simulink model "testrig_Sedan_Hamba_Parts"  (R2026a)
settings: Solver=VariableStepAuto
model workspace (MAT data in the model file):
  smiData : object (value not decoded)
undefined symbols (not defined in the file): Visual, X, Y, Z
libraries: sm_lib x9, Sedan_Hamba_Parts x5, Driver_Human x1, nesl_utility x1, SteeringWheel_Sedan x1
Description:
  | Copyright 2020-2026 The MathWorks, Inc.
settings Model: Creator=smiller  LastModifiedBy=smiller
settings DataIOCC: SignalLoggingName=logsout_testrig_Sedan_Hamba_Parts
settings SimscapeCC: SimscapeNominalValues="[{\"value\":\"1\",\"unit\":\"A\"},{\"value\":\"1\",\"unit\":\"bar\"},{\"value\":\"1\",\"unit\":\"cm^2\"},{\"value\":\"1\",\"unit\":\"cm^3/s\"},{\"value\":\"1\",\"unit\":\"kJ/kg\"},{\"value\":\"1\",\"unit\":\"kW\"},{\"value\":\"1\",\"unit\":\"l\"},{\"value\":\"1\",\"unit\":\"N\"},{\"value\":\"1\",\"unit\":\"N*m\"},{\"value\":\"1\",\"unit\":\"V\"}]"  SimscapeLogName=simlog_testrig_Sedan_Hamba_Parts  SimscapeLogLimitData=off  SimscapeLogDataHistory=5000.0
settings ExplorerConfigSet: InternalSimMechanicsExplorerSettings="<ExplorerConfiguration><canonicalview>default</canonicalview><AnimationSetting><BasePlaybackSpeed>1.0</BasePlaybackSpeed><PlaybackSpeedFactor>1.0</PlaybackSpeedFactor></AnimationSetting><TilePanel><TileInfo><Tiles Columns=\"4\" Count=\"5\" Rows=\"2\"><Column Weight=\"0.2495\"/><Column Weight=\"0.2502\"/><Column Weight=\"0.2502\"/><Column Weight=\"0.2502\"/><Row Weight=\"0.5\"/><Row Weight=\"0.5\"/><Tile Height=\"1\" Width=\"2\" X=\"0\" Y=\"0\"/><Tile Height=\"1\" Width=\"1\" X=\"0\" Y=\"1\"/><Tile Height=\"1\" Width=\"1\" X=\"1\" Y=\"1\"/><Tile Height=\"2\" Width=\"1\" X=\"2\" Y=\"0\"/><Tile Height=\"2\" Width=\"1\" X=\"3\" Y=\"0\"/></Tiles></TileInfo><SceneInfo><SceneViewer><BGColor><R>1</R><G>1</G><B>1</B></BGColor><Camera><DoPerspective>off</DoPerspective><Position><X>-1.59584137542381477</X><Y>-3.07198027242650129</Y><Z>0.760921289715820848</Z></Position><Center><X>-1.59584137542381477</X><Y>9.83512446665057993e-05</Y><Z>0.760921289715820848</Z></Center><Up><X>0</X><Y>-0</Y><Z>1</Z></Up><ViewLimDist>1</ViewLimDist><YLim>1.54679098136813686</YLim><XLim>2.96180666614913024</XLim></Camera></SceneViewer><SceneViewer><BGColor><R>1</R><G>1</G><B>1</B></BGColor><Camera><DoPerspective>off</DoPerspective><Position><X>-4.60166010005607795</X><Y>9.83517575852133064e-05</Y><Z>0.760921289715820404</Z></Position><Center><X>-1.59584130750632891</X><Y>9.83517575852133064e-05</Y><Z>0.760921289715820404</Z></Center><Up><X>0</X><Y>0</Y><Z>1</Z></Up><ViewLimDist>1</ViewLimDist><YLim>1.31762503572872713</YLim><XLim>1.24813568293167454</XLim></Camera></SceneViewer><SceneViewer><BGColor><R>1</R><G>1</G><B>1</B></BGColor><Camera><DoPerspective>off</DoPerspective><Position><X>1.51881627938604935</X><Y>9.83517575848802394e-05</Y><Z>0.760921289715820626</Z></Position><Center><X>-1.59584130749756814</X><Y>9.83517575848802394e-05</Y><Z>0.760921289715820626</Z></Center><Up><X>-0</X><Y>0</Y><Z>1</Z></Up><ViewLimDist>1</ViewLimDist><YLim>1.3143876277785338</YLim><XLim>1.24773511115690439</XLim></Camera></SceneViewer><SceneViewer><BGColor><R>1</R><G>1</G><B>1</B></BGColor><Camera><DoPerspective>off</DoPerspective><Position><X>-1.59334554123115946</X><Y>0.000480417529161059065</Y><Z>3.92375363925896048</Z></Position><Center><X>-1.59334554123115946</X><Y>0.000480417529161059065</Y><Z>0.760921379127168063</Z></Center><Up><X>0.999987969063779625</X><Y>-0.00490527549658697527</Y><Z>0</Z></Up><ViewLimDist>1</ViewLimDist><YLim>2.68267309636390205</YLim><XLim>1.26180000914402624</XLim></Camera></SceneViewer><SceneViewer><BGColor><R>1</R><G>1</G><B>1</B></BGColor><Camera><DoPerspective>off</DoPerspective><Position><X>-1.59407693110947379</X><Y>0.000371021323444242768</Y><Z>-2.22780257404460524</Z></Position><Center><X>-1.59407693110947379</X><Y>0.000371021323444242768</Y><Z>0.760921180858233459</Z></Center><Up><X>0.999993985084104753</X><Y>-0.0034683995749620368</Y><Z>0</Z></Up><ViewLimDist>1</ViewLimDist><YLim>2.6739205639543937</YLim><XLim>1.25768324013131272</XLim></Camera></SceneViewer></SceneInfo></TilePanel><MechEditorPanel><Cameras/><GfxPanelCameraMap/><VideoCreator><PlaybackSpeedRatio>1.0</PlaybackSpeedRatio><FrameRate>30</FrameRate><VideoFormat>Motion JPEG AVI</VideoFormat><FrameSize>auto</FrameSize></VideoCreator></MechEditorPanel></ExplorerConfiguration>"

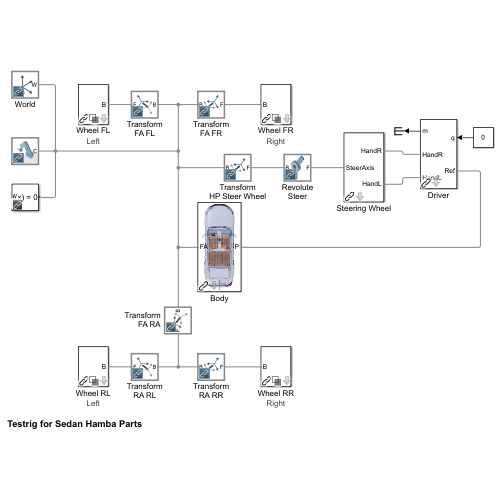
[thumbnail: Simulink's stored preview of the top-level diagram]
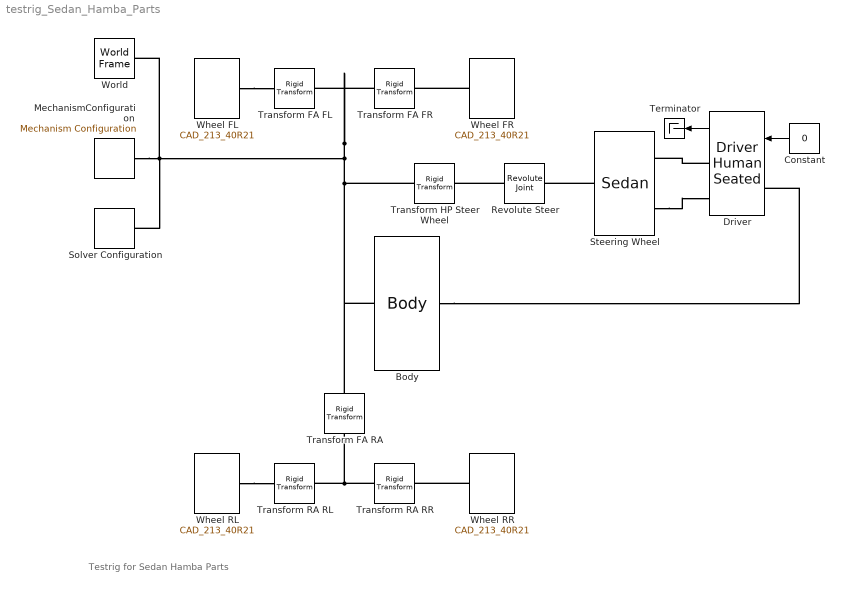
== system testrig_Sedan_Hamba_Parts ==
  note: Testrig for Sedan Hamba Parts
  Body : Sedan_Hamba_Parts/Body  body_clr=VDatabase.BodyGeometry.CAD_Sedan_Hamba.Color.Value  body_opc=VDatabase.BodyGeometry.CAD_Sedan_Hamba.Opacity.Value  glass_opc=BodyGeometry.GlassOpacity.Value  extr_data_emblem_f=Visual.emblem.data*0.2  clr_emblem_f=BodyGeometry.EmblemColor.Value  opc_emblem_f=Visual.emblem.opc
  Constant : Constant  Value=0
  Driver : Driver_Human/Driver Human Seated  VariantControl=Human  hp_human=Vehicle.Chassis.Body.Passenger.FL.s.Value  rpy_human=Vehicle.Chassis.Body.Passenger.FL.a.Value  rho_human=Vehicle.Chassis.Body.Passenger.FL.rho.Value  head_incl_angle=15  clr_human=[0.792156862745098 0.819607843137255 0.933333333333333]  opc_human=1
  MechanismConfiguration : sm_lib/Utilities/Mechanism Configuration  UniformGravity=Constant  GravityVector=[0 -9.80665 0]  GravityVectorUnits=m/s^2  LinearizationDelta=0.001  JointModeTransitionNonlinearIterations=2
  Revolute Steer : sm_lib/Joints/Revolute Joint  JointMode=Normal  CompositeWrenchDir=FollowerOnBase  CompositeWrenchFrame=BaseFrame  SenseConstraintForce=off  SenseConstraintTorque=off  SenseTotalForce=off  SenseTotalTorque=off  PositionTargetSpecify=on  PositionTargetPriority=High  PositionTargetValue=0  PositionTargetValueUnits=deg  VelocityTargetSpecify=off  VelocityTargetPriority=High  VelocityTargetValue=0  VelocityTargetValueUnits=deg/s  EquilibriumPosition=0  EquilibriumPositionUnits=deg  SpringStiffness=0  SpringStiffnessUnits=N*m/deg  DampingCoefficient=0  DampingCoefficientUnits=N*m/(deg/s)  LowerLimitSpecify=off  LowerLimitBound=-90  LowerLimitBoundUnits=deg  LowerLimitStiffness=1e4  LowerLimitStiffnessUnits=N*m/deg  LowerLimitDamping=10  LowerLimitDampingUnits=N*m/(deg/s)  LowerLimitTransitionRegionWidth=0.1  LowerLimitTransitionRegionWidthUnits=deg  UpperLimitSpecify=off  UpperLimitBound=90  UpperLimitBoundUnits=deg  UpperLimitStiffness=1e4  UpperLimitStiffnessUnits=N*m/deg  UpperLimitDamping=10  UpperLimitDampingUnits=N*m/(deg/s)  UpperLimitTransitionRegionWidth=0.1  UpperLimitTransitionRegionWidthUnits=deg  TorqueActuationMode=NoTorque  MotionActuationMode=ComputedMotion  SensePosition=off  SenseVelocity=off  SenseAcceleration=off  SenseTorqueForce=off  SenseLowerLimitTorqueForce=off  SenseUpperLimitTorqueForce=off
  Solver Configuration : nesl_utility/Solver Configuration  PhysicalDomain=network_engine_domain  SubClassName=solver  LeftPortType=input  RightPortType=generic  Tones=[]  Harmonics=[]  SimulateNoise=off  Profile=off  UseLocalSampling=off  EnableSwitchedLinearOptims=on  FrequencyDomain=off  UseCCode=off  RelTol=0.001  AbsTol=1e-06  MinStep=1e-09  ToWorkspace=off  RevertToSquareIcSolve=off  NumHomotopyIterations=100  PhasorMode=off  PhasorModeNumHarmonics=1  ConsistencySolver=NEWTON_FTOL  CanonicalOrdering=UNORDERED  OptimizeIntermediates=UNOPTIMIZED  IndexReductionMethod=DerivativeReplacement  DoDC=off  ResidualTolerance=1e-09  ConsistencyTolSource=GLOBAL  ConsistencyAbsTol=0.001  ConsistencyRelTol=0.001  ConsistencyTolFactor=0.001  UseLocalSolver=off  LocalSolverChoice=NE_BACKWARD_EULER_ADVANCER  ResolveIndetEquations=on  FunctionEvalNumThread=1  LocalSolverSampleTime=0.001  DoFixedCost=off  MaxNonlinIter=3  MaxModeIter=2  ComputeImpulses=off  ImpulseIterations=2  LinearAlgebra=auto  LinearAlgebraNumThread=0  EquationFormulation=NE_TIME_EF  DelaysMemoryBudget=1024  AutomaticFiltering=on  FilteringTimeConstant=0.001  PartitionStorageMethod=AS_NEEDED  PartitionMemoryBudget=1024  PartitionMethod=FAST  MultibodyUseLocalSolver=off  MultibodyLocalSolverChoice=ODE1  MultibodyLocalSolverSampleTime=0.001
  Steering Wheel : SteeringWheel_Sedan/Sedan  clr_wheel=Visual.SteeringWheel.clr  opc_wheel=1
  Terminator : Terminator
  Transform FA FL : sm_lib/Frames and Transforms/Rigid Transform  RotationMethod=AlignedAxes  FollAlignAxisA=+Z  BaseAlignAxisA=+Y  FollAlignAxisB=+Y  BaseAlignAxisB=+Z  RotationStandardAxis=+Z  RotationAngle=0  RotationAngleUnits=deg  RotationArbitraryAxis=[0 0 1]  RotationSequenceAxes=FollowerAxes  RotationSequence=XYX  RotationSequenceAngles=[0 0 0]  RotationSequenceAnglesUnits=deg  RotationMatrix=[1 0 0; 0 1 0; 0 0 1]  Quaternion=[1 0 0 0]  TranslationMethod=Cartesian  TranslationCartesianOffset=[0.00042233863921 0.758005532558466 0.348838382283903]  TranslationCartesianOffsetUnits=m  TranslationStandardAxis=+Z  TranslationStandardOffset=0  TranslationStandardOffsetUnits=m  TranslationROffset=0  TranslationROffsetUnits=m  TranslationThetaOffset=0  TranslationThetaOffsetUnits=deg  TranslationZOffset=0  TranslationZOffsetUnits=m
  Transform FA FR : sm_lib/Frames and Transforms/Rigid Transform  RotationMethod=AlignedAxes  FollAlignAxisA=+Z  BaseAlignAxisA=+Y  FollAlignAxisB=+Y  BaseAlignAxisB=+Z  RotationStandardAxis=+Z  RotationAngle=0  RotationAngleUnits=deg  RotationArbitraryAxis=[0 0 1]  RotationSequenceAxes=FollowerAxes  RotationSequence=XYX  RotationSequenceAngles=[0 0 0]  RotationSequenceAnglesUnits=deg  RotationMatrix=[1 0 0; 0 1 0; 0 0 1]  Quaternion=[1 0 0 0]  TranslationMethod=Cartesian  TranslationCartesianOffset=[0.00042233863921 -0.758005532558466 0.348838382283903]  TranslationCartesianOffsetUnits=m  TranslationStandardAxis=+Z  TranslationStandardOffset=0  TranslationStandardOffsetUnits=m  TranslationROffset=0  TranslationROffsetUnits=m  TranslationThetaOffset=0  TranslationThetaOffsetUnits=deg  TranslationZOffset=0  TranslationZOffsetUnits=m
  Transform FA RA : sm_lib/Frames and Transforms/Rigid Transform  RotationMethod=None  FollAlignAxisA=+X  BaseAlignAxisA=+Y  FollAlignAxisB=+Y  BaseAlignAxisB=+Z  RotationStandardAxis=+Z  RotationAngle=0  RotationAngleUnits=deg  RotationArbitraryAxis=[0 0 1]  RotationSequenceAxes=FollowerAxes  RotationSequence=XYX  RotationSequenceAngles=[0 0 0]  RotationSequenceAnglesUnits=deg  RotationMatrix=[1 0 0; 0 1 0; 0 0 1]  Quaternion=[1 0 0 0]  TranslationMethod=Cartesian  TranslationCartesianOffset=[-2.82158221375407 0 0]  TranslationCartesianOffsetUnits=m  TranslationStandardAxis=+Z  TranslationStandardOffset=0  TranslationStandardOffsetUnits=m  TranslationROffset=0  TranslationROffsetUnits=m  TranslationThetaOffset=0  TranslationThetaOffsetUnits=deg  TranslationZOffset=0  TranslationZOffsetUnits=m
  Transform HP Steer Wheel : sm_lib/Frames and Transforms/Rigid Transform  RotationMethod=StandardAxis  FollAlignAxisA=+X  BaseAlignAxisA=+Y  FollAlignAxisB=+Y  BaseAlignAxisB=+Z  RotationStandardAxis=+Y  RotationAngle=-69.781883336351  RotationAngleUnits=deg  RotationArbitraryAxis=[0 0 1]  RotationSequenceAxes=FollowerAxes  RotationSequence=XYX  RotationSequenceAngles=[0 0 0]  RotationSequenceAnglesUnits=deg  RotationMatrix=[1 0 0; 0 1 0; 0 0 1]  Quaternion=[1 0 0 0]  TranslationMethod=Cartesian  TranslationCartesianOffset=[-1.0213531220517 0.376755175037545 0.923261538853403]  TranslationCartesianOffsetUnits=m  TranslationStandardAxis=+Z  TranslationStandardOffset=0  TranslationStandardOffsetUnits=m  TranslationROffset=0  TranslationROffsetUnits=m  TranslationThetaOffset=0  TranslationThetaOffsetUnits=deg  TranslationZOffset=0  TranslationZOffsetUnits=m
  Transform RA RL : sm_lib/Frames and Transforms/Rigid Transform  RotationMethod=AlignedAxes  FollAlignAxisA=+Z  BaseAlignAxisA=+Y  FollAlignAxisB=+Y  BaseAlignAxisB=+Z  RotationStandardAxis=+Z  RotationAngle=0  RotationAngleUnits=deg  RotationArbitraryAxis=[0 0 1]  RotationSequenceAxes=FollowerAxes  RotationSequence=XYX  RotationSequenceAngles=[0 0 0]  RotationSequenceAnglesUnits=deg  RotationMatrix=[1 0 0; 0 1 0; 0 0 1]  Quaternion=[1 0 0 0]  TranslationMethod=Cartesian  TranslationCartesianOffset=[0.00042233863921 0.758005532558466 0.348838382283903]  TranslationCartesianOffsetUnits=m  TranslationStandardAxis=+Z  TranslationStandardOffset=0  TranslationStandardOffsetUnits=m  TranslationROffset=0  TranslationROffsetUnits=m  TranslationThetaOffset=0  TranslationThetaOffsetUnits=deg  TranslationZOffset=0  TranslationZOffsetUnits=m
  Transform RA RR : sm_lib/Frames and Transforms/Rigid Transform  RotationMethod=AlignedAxes  FollAlignAxisA=+Z  BaseAlignAxisA=+Y  FollAlignAxisB=+Y  BaseAlignAxisB=+Z  RotationStandardAxis=+Z  RotationAngle=0  RotationAngleUnits=deg  RotationArbitraryAxis=[0 0 1]  RotationSequenceAxes=FollowerAxes  RotationSequence=XYX  RotationSequenceAngles=[0 0 0]  RotationSequenceAnglesUnits=deg  RotationMatrix=[1 0 0; 0 1 0; 0 0 1]  Quaternion=[1 0 0 0]  TranslationMethod=Cartesian  TranslationCartesianOffset=[0.00042233863921 -0.758005532558466 0.348838382283903]  TranslationCartesianOffsetUnits=m  TranslationStandardAxis=+Z  TranslationStandardOffset=0  TranslationStandardOffsetUnits=m  TranslationROffset=0  TranslationROffsetUnits=m  TranslationThetaOffset=0  TranslationThetaOffsetUnits=deg  TranslationZOffset=0  TranslationZOffsetUnits=m
  Wheel FL : Sedan_Hamba_Parts/CAD_213_40R21  LabelModeActiveChoice=Left  popup_leftRight=Left  mass_tire=10  mass_rim=0  tire_inertia=[1 2]  rim_inertia=[0 0]  offset_cg=[0 0 0]
      settings: AttributesFormatString=%<LabelModeActiveChoice>
  Wheel FR : Sedan_Hamba_Parts/CAD_213_40R21  LabelModeActiveChoice=Right  popup_leftRight=Right  mass_tire=10  mass_rim=0  tire_inertia=[1 2]  rim_inertia=[0 0]  offset_cg=[0 0 0]
      settings: AttributesFormatString=%<LabelModeActiveChoice>
  Wheel RL : Sedan_Hamba_Parts/CAD_213_40R21  LabelModeActiveChoice=Left  popup_leftRight=Left  mass_tire=10  mass_rim=0  tire_inertia=[1 2]  rim_inertia=[0 0]  offset_cg=[0 0 0]
      settings: AttributesFormatString=%<LabelModeActiveChoice>
  Wheel RR : Sedan_Hamba_Parts/CAD_213_40R21  LabelModeActiveChoice=Right  popup_leftRight=Right  mass_tire=10  mass_rim=0  tire_inertia=[1 2]  rim_inertia=[0 0]  offset_cg=[0 0 0]
      settings: AttributesFormatString=%<LabelModeActiveChoice>
  World : sm_lib/Frames and Transforms/World Frame
  wires:
  Driver/1 -> Terminator/1
  Constant/1 -> Driver/1
  connections:
  Wheel FL/LConn1 -- Transform FA FL/RConn1
  Wheel FR/LConn1 -- Transform FA FR/RConn1
  Wheel RL/LConn1 -- Transform RA RL/RConn1
  Wheel RR/LConn1 -- Transform RA RR/RConn1
  Transform RA RR/LConn1 -- Transform RA RL/LConn1 -- Transform FA RA/RConn1
  Steering Wheel/LConn1 -- Revolute Steer/RConn1
  Revolute Steer/LConn1 -- Transform HP Steer Wheel/RConn1
  MechanismConfiguration/RConn1 -- World/RConn1 -- Transform FA RA/LConn1 -- Body/RConn1 -- Transform HP Steer Wheel/LConn1 -- Transform FA FR/LConn1 -- Transform FA FL/LConn1 -- Solver Configuration/RConn1
  Driver/RConn1 -- Steering Wheel/RConn1
  Steering Wheel/RConn2 -- Driver/RConn2
  Body/LConn1 -- Driver/LConn1
